simulink model "wayPoint"  (R2017a)
settings: Solver=FixedStepAuto  StartTime=0.0  StopTime=240  FixedStep=0.2  RelTol=1e-3
libraries: simulink x1
settings Model: Creator=acrab  LastModifiedBy=acrab

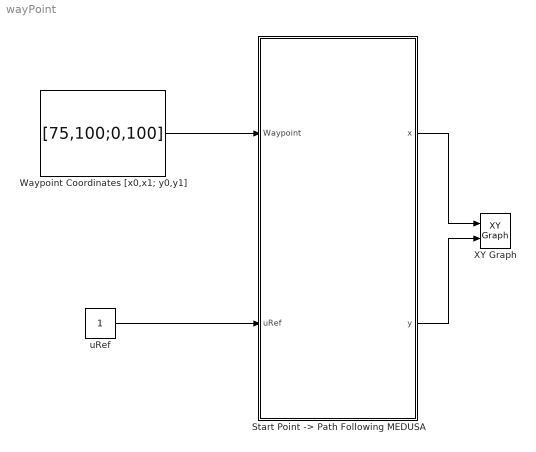
== system wayPoint ==
  "Start Point -> Path Following MEDUSA" : Subsystem
  Waypoint Coordinates [x0,x1; y0,y1] : Constant  Value=[75,100;0,100]
  XY Graph : simulink/Sinks/XY Graph  xmin=-240  xmax=240  ymin=-240  ymax=240  st=-1
  uRef : Constant
  wires:
  Waypoint Coordinates [x0,x1; y0,y1]/1 -> "Start Point -> Path Following MEDUSA"/1(Waypoint)
  uRef/1 -> "Start Point -> Path Following MEDUSA"/2(uRef)
  "Start Point -> Path Following MEDUSA"/1(x) -> XY Graph/1
  "Start Point -> Path Following MEDUSA"/2(y) -> XY Graph/2

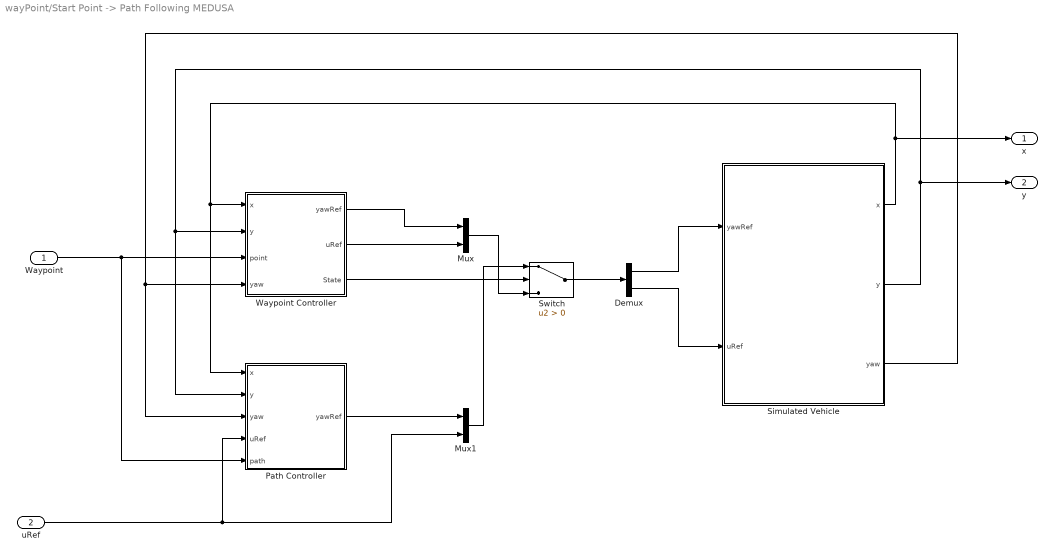
== system wayPoint/Start Point -> Path Following MEDUSA ==
  Waypoint : Inport
  uRef : Inport  Port=2
  Demux : Demux  Outputs=2
  Mux : Mux  Inputs=2
  Mux1 : Mux  Inputs=2
  Path Controller : Subsystem
  Simulated Vehicle : Subsystem
  Switch : Switch  Criteria=u2 > Threshold
  Waypoint Controller : Subsystem  mask{ku=0.5, ks=0.1}
  x : Outport
  y : Outport  Port=2
  wires:
  Waypoint/1 -> Path Controller/5(path), Waypoint Controller/3("point ")
  Waypoint Controller/2(uRef) -> Mux/2
  Switch/1 -> Demux/1
  Path Controller/1(yawRef) -> Mux1/1
  Waypoint Controller/1(yawRef) -> Mux/1
  uRef/1 -> Path Controller/4(uRef), Mux1/2
  Waypoint Controller/3(State) -> Switch/2
  Mux/1 -> Switch/3
  Demux/1 -> Simulated Vehicle/1(yawRef)
  Mux1/1 -> Switch/1
  Simulated Vehicle/2(y) -> Waypoint Controller/2("y "), Path Controller/2("y "), y/1
  Demux/2 -> Simulated Vehicle/2(uRef)
  Simulated Vehicle/3(yaw) -> Waypoint Controller/4(yaw), Path Controller/3(yaw)
  Simulated Vehicle/1(x) -> x/1, Path Controller/1(x), Waypoint Controller/1(x)

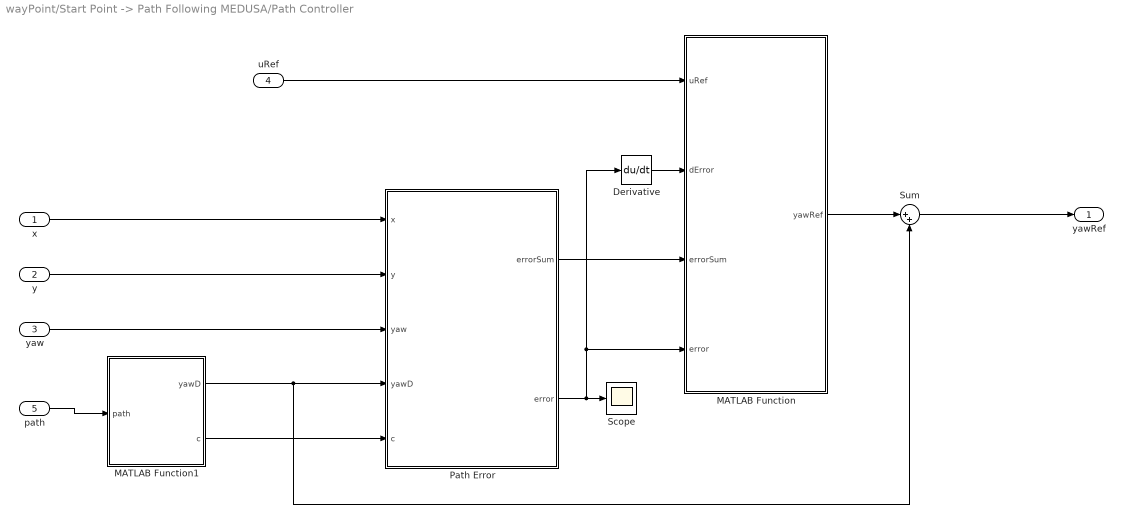
== system wayPoint/Start Point -> Path Following MEDUSA/Path Controller ==
  x : Inport
  "y " : Inport  Port=2
  yaw : Inport  Port=3
  uRef : Inport  Port=4
  path : Inport  Port=5
  Derivative : Derivative
  MATLAB Function : MATLAB Function  TreatAsAtomicUnit=on
  MATLAB Function1 : MATLAB Function  TreatAsAtomicUnit=on
  Path Error : MATLAB Function  TreatAsAtomicUnit=on
  Scope : Scope
  Sum : Sum  Inputs=|++
  yawRef : Outport
  wires:
  path/1 -> MATLAB Function1/1(path)
  Sum/1 -> yawRef/1
  MATLAB Function/1(yawRef) -> Sum/1
  Derivative/1 -> MATLAB Function/2(dError)
  uRef/1 -> MATLAB Function/1(uRef)
  yaw/1 -> Path Error/3(yaw)
  MATLAB Function1/1(yawD) -> Path Error/4(yawD), Sum/2
  "y "/1 -> Path Error/2(y)
  Path Error/2(error) -> Scope/1, MATLAB Function/4(error), Derivative/1
  MATLAB Function1/2(c) -> Path Error/5(c)
  x/1 -> Path Error/1(x)
  Path Error/1(errorSum) -> MATLAB Function/3(errorSum)

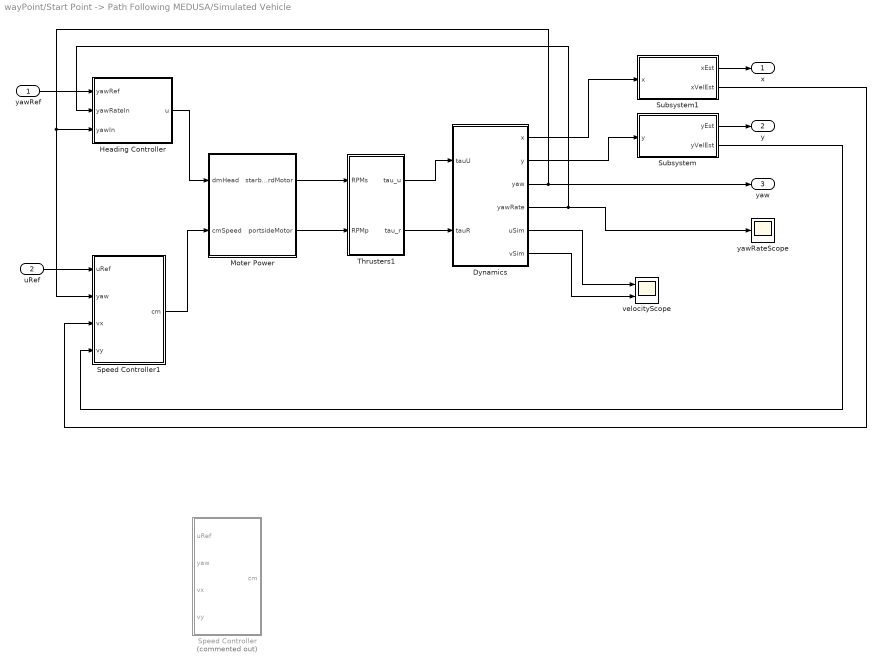
== system wayPoint/Start Point -> Path Following MEDUSA/Simulated Vehicle ==
  yawRef : Inport
  uRef : Inport  Port=2
  Dynamics : Subsystem
  Heading Controller : Subsystem  mask{Kp=45, Kd=110}
  Moter Power : Subsystem
  Speed Controller : Subsystem  Commented=on  mask{Kp=60, Ki=-2}
  Speed Controller1 : Subsystem  mask{Kp=60, Ki=3, KSat=60}
      mask prompts: KSat "Saturation Level"
  Subsystem : Subsystem
  Subsystem1 : Subsystem
  Thrusters1 : Subsystem
  velocityScope : Scope  NumInputPorts=2
  yawRateScope : Scope
  x : Outport
  y : Outport  Port=2
  yaw : Outport  Port=3
  wires:
  Thrusters1/1(tau_u) -> Dynamics/1(tauU)
  Thrusters1/2(tau_r) -> Dynamics/2(tauR)
  Moter Power/1(starboardMotor) -> Thrusters1/1(RPMs)
  Moter Power/2(portsideMotor) -> Thrusters1/2(RPMp)
  Dynamics/3(yaw) -> Speed Controller1/2(yaw), Heading Controller/3(yawIn), yaw/1
  Dynamics/4(yawRate) -> yawRateScope/1, Heading Controller/2(yawRateIn)
  Dynamics/5(uSim) -> velocityScope/1
  Dynamics/6(vSim) -> velocityScope/2
  yawRef/1 -> Heading Controller/1(yawRef)
  uRef/1 -> Speed Controller1/1(uRef)
  Subsystem/1(yEst) -> y/1
  Dynamics/2(y) -> Subsystem/1(y)
  Heading Controller/1(u) -> Moter Power/1(dmHead)
  Speed Controller1/1(cm) -> Moter Power/2(cmSpeed)
  Dynamics/1(x) -> Subsystem1/1(x)
  Subsystem1/1(xEst) -> x/1
  Subsystem/2(yVelEst) -> Speed Controller1/4(vy)
  Subsystem1/2(xVelEst) -> Speed Controller1/3(vx)

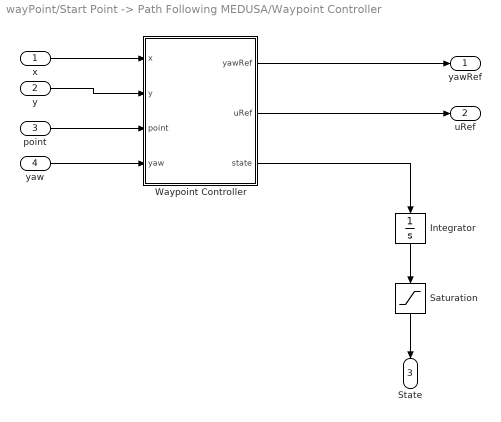
== system wayPoint/Start Point -> Path Following MEDUSA/Waypoint Controller ==
  x : Inport
  "y " : Inport  Port=2
  "point " : Inport  Port=3
  yaw : Inport  Port=4
  Integrator : Integrator
  Saturation : Saturate  UpperLimit=1  LowerLimit=0
  Waypoint Controller : MATLAB Function  TreatAsAtomicUnit=on
  yawRef : Outport
  uRef : Outport  Port=2
  State : Outport  Port=3
  wires:
  x/1 -> Waypoint Controller/1(x)
  Waypoint Controller/2(uRef) -> uRef/1
  "point "/1 -> Waypoint Controller/3(point)
  Waypoint Controller/1(yawRef) -> yawRef/1
  "y "/1 -> Waypoint Controller/2(y)
  yaw/1 -> Waypoint Controller/4(yaw)
  Waypoint Controller/3(state) -> Integrator/1
  Integrator/1 -> Saturation/1
  Saturation/1 -> State/1

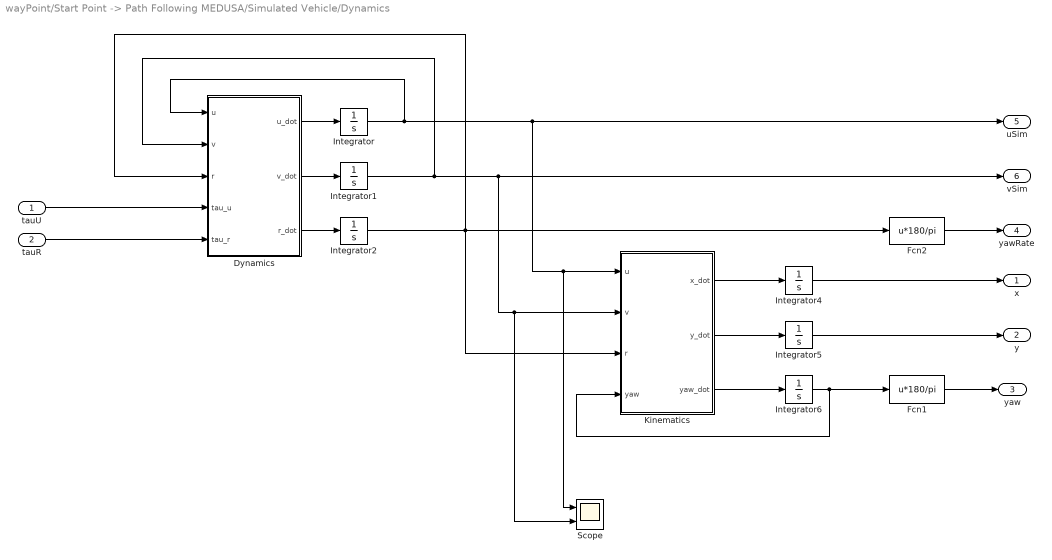
== system wayPoint/Start Point -> Path Following MEDUSA/Simulated Vehicle/Dynamics ==
  tauU : Inport
  tauR : Inport  Port=2
  Dynamics : MATLAB Function  TreatAsAtomicUnit=on
  Fcn1 : Fcn  Expr=u*180/pi
  Fcn2 : Fcn  Expr=u*180/pi
  Integrator{,1..2,4..6} (6 alike) : Integrator
  Kinematics : MATLAB Function  TreatAsAtomicUnit=on
  Scope : Scope  NumInputPorts=2
  x : Outport
  y : Outport  Port=2
  yaw : Outport  Port=3
  yawRate : Outport  Port=4
  uSim : Outport  Port=5
  vSim : Outport  Port=6
  wires:
  tauR/1 -> Dynamics/5(tau_r)
  tauU/1 -> Dynamics/4(tau_u)
  Dynamics/1(u_dot) -> Integrator/1
  Dynamics/3(r_dot) -> Integrator2/1
  Dynamics/2(v_dot) -> Integrator1/1
  Kinematics/1(x_dot) -> Integrator4/1
  Kinematics/2(y_dot) -> Integrator5/1
  Kinematics/3(yaw_dot) -> Integrator6/1
  Integrator/1 -> uSim/1, Scope/1, Kinematics/1(u), Dynamics/1(u)
  Integrator1/1 -> vSim/1, Kinematics/2(v), Scope/2, Dynamics/2(v)
  Integrator2/1 -> Fcn2/1, Kinematics/3(r), Dynamics/3(r)
  Integrator4/1 -> x/1
  Integrator5/1 -> y/1
  Integrator6/1 -> Fcn1/1, Kinematics/4(yaw)
  Fcn1/1 -> yaw/1
  Fcn2/1 -> yawRate/1

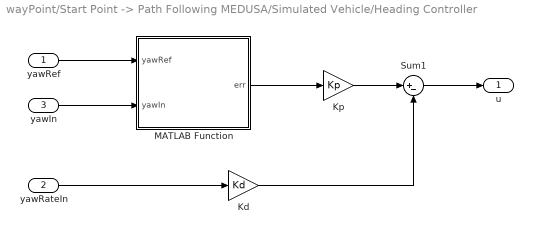
== system wayPoint/Start Point -> Path Following MEDUSA/Simulated Vehicle/Heading Controller ==
  yawRef : Inport
  yawRateIn : Inport  Port=2
  yawIn : Inport  Port=3
  Kd : Gain  Gain=Kd
  Kp : Gain  Gain=Kp
  MATLAB Function : MATLAB Function  TreatAsAtomicUnit=on
  Sum1 : Sum  Inputs=|+-
  u : Outport
  wires:
  yawRef/1 -> MATLAB Function/1(yawRef)
  yawRateIn/1 -> Kd/1
  Kd/1 -> Sum1/2
  Kp/1 -> Sum1/1
  Sum1/1 -> u/1
  MATLAB Function/1(err) -> Kp/1
  yawIn/1 -> MATLAB Function/2(yawIn)

== system wayPoint/Start Point -> Path Following MEDUSA/Simulated Vehicle/Moter Power ==
  dmHead : Inport
  cmSpeed : Inport  Port=2
  MATLAB Function : MATLAB Function  TreatAsAtomicUnit=on
  starboardMotor : Outport
  portsideMotor : Outport  Port=2
  wires:
  dmHead/1 -> MATLAB Function/1(dmHead)
  cmSpeed/1 -> MATLAB Function/2(cmSpeed)
  MATLAB Function/1(Pm) -> portsideMotor/1
  MATLAB Function/2(Sm) -> starboardMotor/1

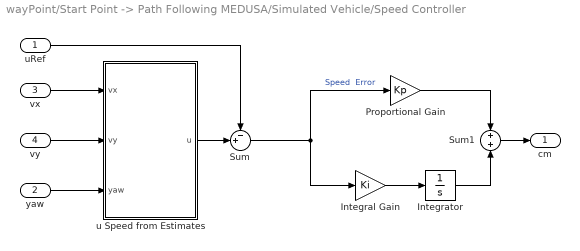
== system wayPoint/Start Point -> Path Following MEDUSA/Simulated Vehicle/Speed Controller ==
  uRef : Inport
  yaw : Inport  Port=2
  vx : Inport  Port=3
  vy : Inport  Port=4
  Integral Gain : Gain  Gain=Ki
  Integrator : Integrator
  Proportional Gain : Gain  Gain=Kp
  Sum : Sum  Inputs=-+|
  Sum1 : Sum  Inputs=+|+
  u Speed from Estimates : MATLAB Function  TreatAsAtomicUnit=on
  cm : Outport
  wires:
  vx/1 -> u Speed from Estimates/1(vx)
  yaw/1 -> u Speed from Estimates/3(yaw)
  vy/1 -> u Speed from Estimates/2(vy)
  uRef/1 -> Sum/1
  u Speed from Estimates/1(u) -> Sum/2
  Sum/1 -> Integral Gain/1, Proportional Gain/1  "Speed  Error"
  Integral Gain/1 -> Integrator/1
  Proportional Gain/1 -> Sum1/1
  Integrator/1 -> Sum1/2
  Sum1/1 -> cm/1

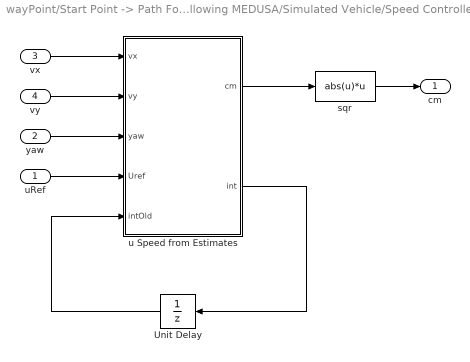
== system wayPoint/Start Point -> Path Following MEDUSA/Simulated Vehicle/Speed Controller1 ==
  uRef : Inport
  yaw : Inport  Port=2
  vx : Inport  Port=3
  vy : Inport  Port=4
  Unit Delay : UnitDelay  SampleTime=-1
  sqr : Fcn  Expr=abs(u)*u
  u Speed from Estimates : MATLAB Function  TreatAsAtomicUnit=on
  cm : Outport
  wires:
  vx/1 -> u Speed from Estimates/1(vx)
  yaw/1 -> u Speed from Estimates/3(yaw)
  vy/1 -> u Speed from Estimates/2(vy)
  uRef/1 -> u Speed from Estimates/4(Uref)
  sqr/1 -> cm/1
  Unit Delay/1 -> u Speed from Estimates/5(intOld)
  u Speed from Estimates/1(cm) -> sqr/1
  u Speed from Estimates/2(int) -> Unit Delay/1

== system wayPoint/Start Point -> Path Following MEDUSA/Simulated Vehicle/Subsystem ==
  y : Inport
  Derivative : Derivative
  yEst : Outport
  yVelEst : Outport  Port=2
  wires:
  y/1 -> Derivative/1, yEst/1
  Derivative/1 -> yVelEst/1

== system wayPoint/Start Point -> Path Following MEDUSA/Simulated Vehicle/Subsystem1 ==
  x : Inport
  Derivative : Derivative
  xEst : Outport
  xVelEst : Outport  Port=2
  wires:
  x/1 -> Derivative/1, xEst/1
  Derivative/1 -> xVelEst/1

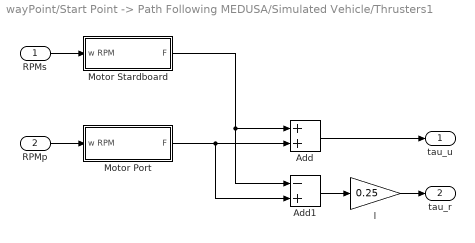
== system wayPoint/Start Point -> Path Following MEDUSA/Simulated Vehicle/Thrusters1 ==
  RPMs : Inport
  RPMp : Inport  Port=2
  Add : Sum
  Add1 : Sum  Inputs=-+
  Motor Port : Subsystem  mask{K0=7.2115, tau=0.346, eta=4/(1500^2)}
      mask prompts: tau "Atraso do Motor"; eta "Constante de conversao W-F"
  Motor Stardboard : Subsystem  mask{K0=7.2115, tau=0.346, eta=4/(1500^2)}
      mask prompts: tau "Atraso do Motor"; eta "Constante de conversao W-F"
  l : Gain  Gain=0.25
  tau_u : Outport
  tau_r : Outport  Port=2
  wires:
  Add1/1 -> l/1
  RPMs/1 -> Motor Stardboard/1(w RPM)
  Add/1 -> tau_u/1
  RPMp/1 -> Motor Port/1(w RPM)
  l/1 -> tau_r/1
  Motor Port/1(F) -> Add/2, Add1/2
  Motor Stardboard/1(F) -> Add/1, Add1/1

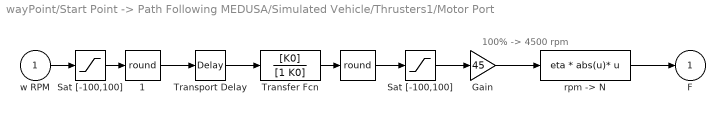
== system wayPoint/Start Point -> Path Following MEDUSA/Simulated Vehicle/Thrusters1/Motor Port ==
  note: 100% -> 4500 rpm
  w RPM : Inport
  "  " : Rounding  Operator=round
  "  1" : Rounding  Operator=round
  Gain : Gain  Gain=45
  Sat [-100,100] : Saturate  UpperLimit=100  LowerLimit=-100
  "Sat [-100,100] " : Saturate  UpperLimit=100  LowerLimit=-100
  Transfer Fcn : TransferFcn  Numerator=[K0]  Denominator=[1 K0]
  Transport Delay : TransportDelay  DelayTime=tau
  "rpm -> N" : Fcn  Expr=eta * abs(u)* u
  F : Outport
  wires:
  Transfer Fcn/1 -> "  "/1
  Transport Delay/1 -> Transfer Fcn/1
  "  1"/1 -> Transport Delay/1
  "  "/1 -> "Sat [-100,100] "/1
  "rpm -> N"/1 -> F/1
  Sat [-100,100]/1 -> "  1"/1
  Gain/1 -> "rpm -> N"/1
  w RPM/1 -> Sat [-100,100]/1
  "Sat [-100,100] "/1 -> Gain/1

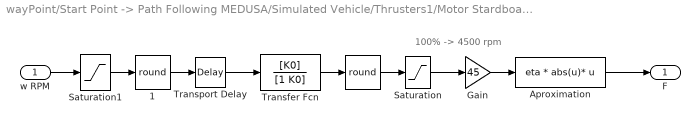
== system wayPoint/Start Point -> Path Following MEDUSA/Simulated Vehicle/Thrusters1/Motor Stardboard ==
  note: 100% -> 4500 rpm
  w RPM : Inport
  "  " : Rounding  Operator=round
  "  1" : Rounding  Operator=round
  Aproximation : Fcn  Expr=eta * abs(u)* u
  Gain : Gain  Gain=45
  Saturation : Saturate  UpperLimit=100  LowerLimit=-100
  Saturation1 : Saturate  UpperLimit=100  LowerLimit=-100
  Transfer Fcn : TransferFcn  Numerator=[K0]  Denominator=[1 K0]
  Transport Delay : TransportDelay  DelayTime=tau
  F : Outport
  wires:
  Transfer Fcn/1 -> "  "/1
  Transport Delay/1 -> Transfer Fcn/1
  "  1"/1 -> Transport Delay/1
  "  "/1 -> Saturation/1
  Aproximation/1 -> F/1
  Saturation1/1 -> "  1"/1
  Gain/1 -> Aproximation/1
  w RPM/1 -> Saturation1/1
  Saturation/1 -> Gain/1

== matlab function wayPoint/Start Point -> Path Following MEDUSA/Simulated Vehicle/Dynamics/Dynamics ==
  data: u input; u_dot output; v input; r input; tau_u input; tau_r input; v_dot output; r_dot output
function [u_dot,v_dot,r_dot] = fcn(u,v,r,tau_u,tau_r)

% Coefficients
m = 17; %kg
Iz = 1; %4.14;
X_u_dot = -20;
Y_v_dot = -30;%-1.3175;
N_r_dot = -8.69;% -0.5;
X_u = -0.2;
Y_v = -50; %-55.117;
N_r = -4.14; %-0.1
X_uu = -25;
Y_vv = -0.01;%-101.2776;
N_rr = -6.23; %-21

% Added Mass
mu = m - X_u_dot;
mv = m - Y_v_dot;
mr = Iz - N_r_dot;
muv = mu - mv;

% Hydrodynamic Damping
du = - X_u - X_uu*abs(u);
dv = - Y_v - Y_vv*abs(v);
dr = - N_r - N_rr*abs(r);

% State Derivatives
u_dot = 1/mu*(tau_u + mv*v*r - du*u);
v_dot = 1/mv*(- mu*u*r - dv*v);
r_dot = 1/mr*(tau_r + muv*u*v - dr*r);

== matlab function wayPoint/Start Point -> Path Following MEDUSA/Waypoint Controller/Waypoint Controller ==
  data: yawRef output; x input; y input; uRef output; point input; yaw input; state output; ku parameter; ks parameter
function [yawRef, uRef, state] = wayPoint(x,y, point, yaw, ku, ks)
    state = 0;
    % margin
    e = 0.1;
    
    % extract information
    x0 = point(1,1);
    y0 = point(2,1);
    x1 = point(1,2);
    y1 = point(2,2);
    
    % distance to waypoint
    d = sqrt((x - x0)^2 + (y - y0)^2);
    
    % decide on action
    if (d < e)
        state = 1;
        uRef = 0;
        yawRef = atan2d((y1-y0),(x1-x0));

%         point towards next point
%         yawRef = atand((y1-y0)/(x1-x0));
%         yawErr = yawRef - yaw;
%         if (abs(yawErr) < 20)
%             state = 1;
%         end
    else
        uRef = ku*asin(d /(abs(d)+ks))*2/pi;
        % note: yawRef = -atan2d + 90
        yawRef = atan2d((y0-y),(x0-x));
    end
   
end

== matlab function wayPoint/Start Point -> Path Following MEDUSA/Simulated Vehicle/Dynamics/Kinematics ==
  data: u input; x_dot output; v input; r input; yaw input; y_dot output; yaw_dot output
function [x_dot,y_dot,yaw_dot] = fcn(u,v,r,yaw)

x_dot = u*cos(yaw) - v*sin(yaw);
y_dot = u*sin(yaw) + v*cos(yaw);
yaw_dot = r;

== matlab function wayPoint/Start Point -> Path Following MEDUSA/Simulated Vehicle/Moter Power/MATLAB Function ==
  data: dmHead input; cmSpeed input; Pm output; Sm output
function [Pm,Sm] = fcn(dmHead,cmSpeed)

Cm_sqr = cmSpeed;
Dm_sqr = dmHead;

Pm = round(sqrt(abs(Cm_sqr+Dm_sqr))*sign(Cm_sqr+Dm_sqr));
Sm = round(sqrt(abs(Cm_sqr-Dm_sqr))*sign(Cm_sqr-Dm_sqr));

== matlab function wayPoint/Start Point -> Path Following MEDUSA/Simulated Vehicle/Heading Controller/MATLAB Function ==
  data: err output; yawRef input; yawIn input
function err = fcn(yawRef,yawIn)

err = yawRef - yawIn;

if(err>180) 
    
     err = err - 360;
     
elseif(err<-180) 
    
     err = 360 + err;
     
end

== matlab function wayPoint/Start Point -> Path Following MEDUSA/Path Controller/Path Error ==
  data: errorSum output size=2; x input; error output size=2; y input; yaw input; yawD input size=1; c input
% ========================================= %
% Calculating the cross track error between %
% defined path line and current position    %
% ========================================= %

function [errorSum, error]  = pathError(x, y, yaw, yawD,c)

% ARGUMENTS %
% x          current x position
% y          current y position
% m          gradient (for y = mx + c)
% c          y offset (for y = mx + c)

% VARIABLES %
% xD, yD     closest points on line
% error      error in [x, y, yaw]'
% u          vector between desired and real paths 

%extract data
m = tand(yawD);

%function to minimize
    function u = lineDiff(xL)
        u = (xL - x)^2 + (m*xL + c - y)^2;
    end

%desired position
xD = fminbnd(@lineDiff,x-10,x+10);
yD = m*xD + c;
closestPoint = [xD,yD];

%error terms
% difference = [xD-x; yD-y; yawD-yaw];
% trans = rotz(yaw);
% error = trans*difference;

%cross track error
e = sqrt(lineDiff(xD));
if y < (m*x+c)
    e = -e;
end

%yaw error
yawErr = yawD - yaw;

%combine
error = [e;yawErr];

%sum of error
persistent sum;
if isempty(sum)
    sum = [0;0];
end
errorSum = error + sum;
sum = errorSum;


test = [yawD-yaw];
end

== matlab function wayPoint/Start Point -> Path Following MEDUSA/Simulated Vehicle/Speed Controller/u Speed from Estimates ==
  data: vx input; u output; vy input; yaw input
function u = ExtractSpeed(vx,vy,yaw)

u = vx*sind(yaw) + vy*cosd(yaw);


%uBody = 0;

% **VARIABLES**
% T: Transformation matrix, Inertial->Body
% uBody: Current velocity, Body Fixed

%T = [sin(yaw),cos(yaw);cos(yaw),-sin(yaw)];
%uBody = T*[vx;vy];
%u = uBody(1,1);

== matlab function wayPoint/Start Point -> Path Following MEDUSA/Path Controller/MATLAB Function ==
  data: yawRef output; uRef input; dError input; errorSum input; error input
function yawRef  = yawController(uRef, dError, errorSum, error)%K4, K2, K1, K3)

% STEP TIME (REPLACE)
Ts = 0.2;

% Extract Data %
yError     =    error(1,1);
yawError   =    error(2,1);
yError_dot =   dError(1,1);
ySum       = errorSum(1,1);

% Gain Values %
K1 =  1.5; %yaw proportional
K2 = -9.0; %cross-track proportional
K3 =  4.0; %cross-track differential
K4 = -0.05; %integral

% PROVIDE yawRef
yawRef = K1*yawError + K2*yError/uRef ...
         + K3*yError_dot + K4*ySum*Ts;
     
end

== matlab function wayPoint/Start Point -> Path Following MEDUSA/Path Controller/MATLAB Function1 ==
  data: path input; yawD output; c output
function [yawD, c] = fcn(path)
% INPUTS
% n     = vehicle ID no.
% start = [xs1, xs2,...,xsi;
%          ys1, ys2,...,ysi]
% end   = [xe1, xe2,...,xei;
%          ye1, ye2,...,yei]
% for i = {1,..,n} vehicles

% Extract Info
x0 = path(1,1);
y0 = path(2,1);
x1 = path(1,2);
y1 = path(2,2);

% Calculate desired yaw angle
yawD = atand((y1-y0)/(x1-x0));
% Calculate y intersection
c = y0 - tand(yawD)*x0;
end

== matlab function wayPoint/Start Point -> Path Following MEDUSA/Simulated Vehicle/Speed Controller1/u Speed from Estimates ==
  data: vx input; cm output; vy input; yaw input; Uref input; int output; intOld input; Kp parameter; Ki parameter; KSat parameter
function [cm,int] = ExtractSpeed(vx,vy,yaw,Uref,intOld,Kp, Ki, KSat)

% Kp = 60;
% Ki = 2;
% KSat = 60;
 
u = vx*sind(yaw) + vy*cosd(yaw);
err = u - Uref;
int = intOld + err;

cm = - Kp*err - Ki*int;

if(abs(cm) >= KSat)
   cm = KSat*sign(cm); 
   int = intOld;
end
